simulink model "Dead_Zone2"  (R2024a)
settings: Solver=FixedStepAuto  StartTime=0.0  StopTime=10.0  FixedStep=1  RelTol=1e-3
libraries: simulink x2
settings Model: Creator=SAINATH  LastModifiedBy=abhim
settings RTWCC: GPUComputeCapability=3.5

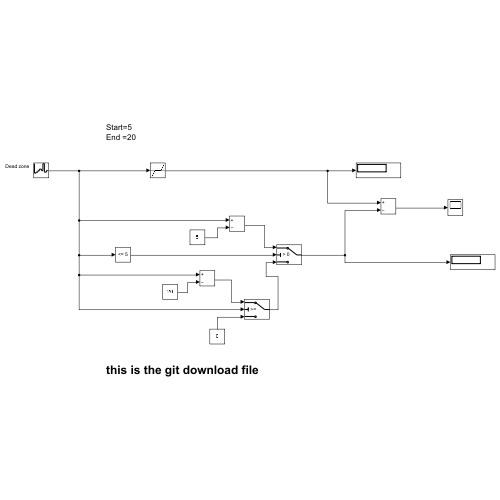
[thumbnail: Simulink's stored preview of the top-level diagram]
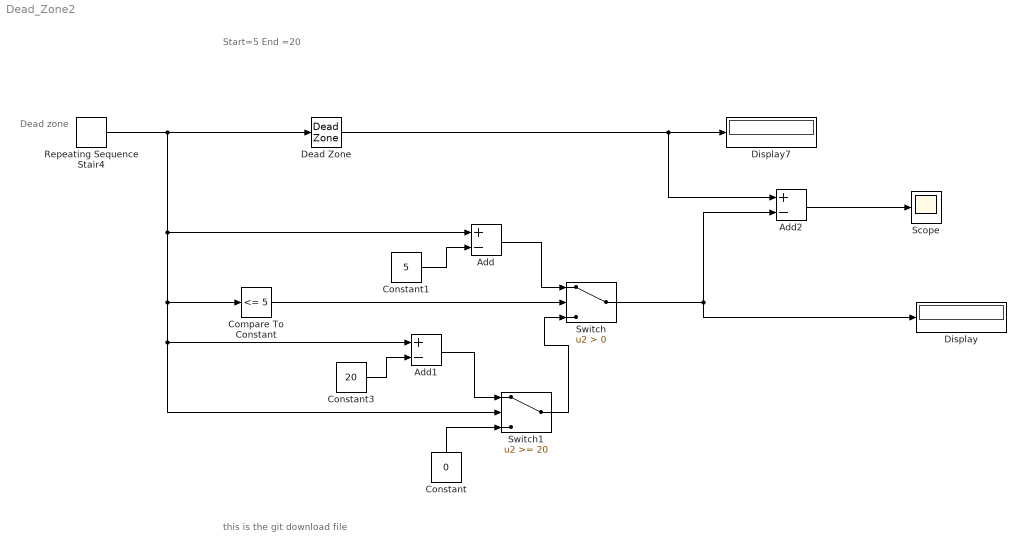
== system Dead_Zone2 ==
  note: this is the git download file
  note: Start=5
      | End =20
  note: Dead zone
  Add : Sum  Inputs=+-
  Add1 : Sum  Inputs=+-
  Add2 : Sum  Inputs=+-
  Compare To Constant : simulink/Logic and Bit Operations/Compare To Constant  relop=<=  const=5  OutDataTypeStr=boolean
  Constant : Constant  Value=0
  Constant1 : Constant  Value=5
  Constant3 : Constant  Value=20
  Dead Zone : DeadZone  LowerValue=5  UpperValue=20
  Display : Display
  Display7 : Display
  Repeating Sequence Stair4 : simulink/Sources/Repeating Sequence Stair  OutValues=[3 11 21 34 23 76 12 22 ].'  tsamp=-1  OutMin=[]  OutMax=[]  OutDataTypeStr=double  OutputDataTypeScalingMode=double  OutDataType=fixdt(0,8)  ConRadixGroup=Best Precision: Vector-wise  OutScaling=2^-12
  Scope : Scope
  Switch : Switch  Criteria=u2 > Threshold  SaturateOnIntegerOverflow=off  InputSameDT=off
  Switch1 : Switch  Threshold=20  SaturateOnIntegerOverflow=off  InputSameDT=off
  wires:
  Dead Zone/1 -> Add2/1, Display7/1
  Constant1/1 -> Add/2
  Constant3/1 -> Add1/2
  Repeating Sequence Stair4/1 -> Compare To Constant/1, Add1/1, Switch1/2, Add/1, Dead Zone/1
  Add/1 -> Switch/1
  Switch/1 -> Add2/2, Display/1
  Add1/1 -> Switch1/1
  Switch1/1 -> Switch/3
  Compare To Constant/1 -> Switch/2
  Constant/1 -> Switch1/3
  Add2/1 -> Scope/1
